simulink model "EHB_speedgoat_R2020a_V1"  (R2020a)
settings: Solver=FixedStepDiscrete  StartTime=0.0  StopTime=inf  FixedStep=0.001  RelTol=1e-3  EnableMultiTasking=on
model workspace (MAT data in the model file):
  A : Simulink.Signal (value not decoded)
  B : Simulink.Signal (value not decoded)
  C : Simulink.Signal (value not decoded)
  D : Simulink.Signal (value not decoded)
  E : Simulink.Signal (value not decoded)
  calin = [-9.96 -7.98 -5.98 -3.99 -1.994 0 1.995 3.992 5.99 7.98 9.97]
  calout = [-10 -8 -6 -4 -2 0 2 4 6 8 10]
symbols that are objects in the model workspace (value not decoded): C, D
undefined symbols (not defined in the file): Com1, none, ts_IO612
libraries: simulink x1436, xpcethercatlib x1223, yisutbxlib_utilities x256, xpcutilitieslib x156, hdlsllib x145, canmsglib x46, speedgoatlib_IO602_4 x11, speedgoatlib_IO611 x7, slrttcplib x4, CanManageLib x3, slrtlib x3, xpcseriallib x2
(part 15 of 30)

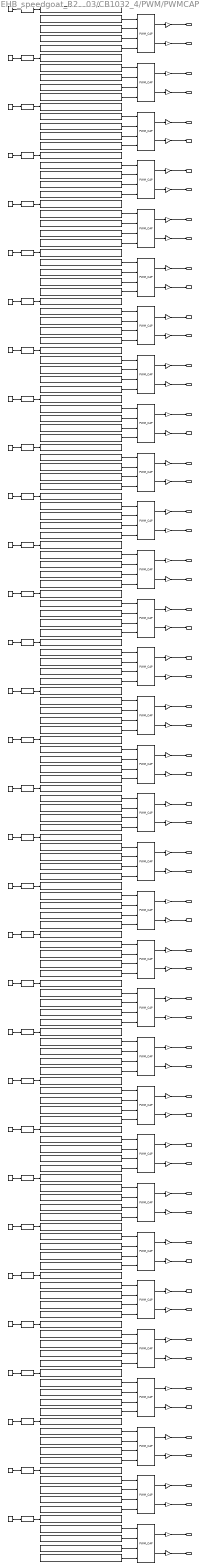
== system EHB_speedgoat_R2020a_V1/保留/TIF_03/CB1032_4/PWM/PWMCAP1 ==
  Constant CPL_CH{1..32} (32 alike) : Constant
  DTCB CPL_CH{1..32} (32 alike) : DataTypeConversion
  Gain_DC_CAP_CH{1..32} (32 alike) : Gain
  Gain_Period_CAP_CH{1..32} (32 alike) : Gain
  PDO Receive HTH_CH1 : xpcethercatlib/EtherCAT PDO Receive  Priority=2  sig_name=Box 4 (YISUWORLD_Dig).PDOGetValue process data mapping.HTH1  sig_offset=8344  sig_type=uint16  type_size=16  sig_dim=1  device_id=0  sample_time=0.001000
      settings: SourceProductBaseCode=XP
  PDO Receive HTH_CH10 : xpcethercatlib/EtherCAT PDO Receive  Priority=2  sig_name=Box 4 (YISUWORLD_Dig).PDOGetValue process data mapping.HTH10  sig_offset=8488  sig_type=uint16  type_size=16  sig_dim=1  device_id=0  sample_time=0.001000
      settings: SourceProductBaseCode=XP
  PDO Receive HTH_CH11 : xpcethercatlib/EtherCAT PDO Receive  Priority=2  sig_name=Box 4 (YISUWORLD_Dig).PDOGetValue process data mapping.HTH11  sig_offset=8504  sig_type=uint16  type_size=16  sig_dim=1  device_id=0  sample_time=0.001000
      settings: SourceProductBaseCode=XP
  PDO Receive HTH_CH12 : xpcethercatlib/EtherCAT PDO Receive  Priority=2  sig_name=Box 4 (YISUWORLD_Dig).PDOGetValue process data mapping.HTH12  sig_offset=8520  sig_type=uint16  type_size=16  sig_dim=1  device_id=0  sample_time=0.001000
      settings: SourceProductBaseCode=XP
  PDO Receive HTH_CH13 : xpcethercatlib/EtherCAT PDO Receive  Priority=2  sig_name=Box 4 (YISUWORLD_Dig).PDOGetValue process data mapping.HTH13  sig_offset=8536  sig_type=uint16  type_size=16  sig_dim=1  device_id=0  sample_time=0.001000
      settings: SourceProductBaseCode=XP
  PDO Receive HTH_CH14 : xpcethercatlib/EtherCAT PDO Receive  Priority=2  sig_name=Box 4 (YISUWORLD_Dig).PDOGetValue process data mapping.HTH14  sig_offset=8552  sig_type=uint16  type_size=16  sig_dim=1  device_id=0  sample_time=0.001000
      settings: SourceProductBaseCode=XP
  PDO Receive HTH_CH15 : xpcethercatlib/EtherCAT PDO Receive  Priority=2  sig_name=Box 4 (YISUWORLD_Dig).PDOGetValue process data mapping.HTH15  sig_offset=8568  sig_type=uint16  type_size=16  sig_dim=1  device_id=0  sample_time=0.001000
      settings: SourceProductBaseCode=XP
  PDO Receive HTH_CH16 : xpcethercatlib/EtherCAT PDO Receive  Priority=2  sig_name=Box 4 (YISUWORLD_Dig).PDOGetValue process data mapping.HTH16  sig_offset=8584  sig_type=uint16  type_size=16  sig_dim=1  device_id=0  sample_time=0.001000
      settings: SourceProductBaseCode=XP
  PDO Receive HTH_CH17 : xpcethercatlib/EtherCAT PDO Receive  Priority=2  sig_name=Box 4 (YISUWORLD_Dig).PDOGetValue process data mapping.HTH17  sig_offset=8600  sig_type=uint16  type_size=16  sig_dim=1  device_id=0  sample_time=0.001000
      settings: SourceProductBaseCode=XP
  PDO Receive HTH_CH18 : xpcethercatlib/EtherCAT PDO Receive  Priority=2  sig_name=Box 4 (YISUWORLD_Dig).PDOGetValue process data mapping.HTH18  sig_offset=8616  sig_type=uint16  type_size=16  sig_dim=1  device_id=0  sample_time=0.001000
      settings: SourceProductBaseCode=XP
  PDO Receive HTH_CH19 : xpcethercatlib/EtherCAT PDO Receive  Priority=2  sig_name=Box 4 (YISUWORLD_Dig).PDOGetValue process data mapping.HTH19  sig_offset=8632  sig_type=uint16  type_size=16  sig_dim=1  device_id=0  sample_time=0.001000
      settings: SourceProductBaseCode=XP
  PDO Receive HTH_CH2 : xpcethercatlib/EtherCAT PDO Receive  Priority=2  sig_name=Box 4 (YISUWORLD_Dig).PDOGetValue process data mapping.HTH2  sig_offset=8360  sig_type=uint16  type_size=16  sig_dim=1  device_id=0  sample_time=0.001000
      settings: SourceProductBaseCode=XP
  PDO Receive HTH_CH20 : xpcethercatlib/EtherCAT PDO Receive  Priority=2  sig_name=Box 4 (YISUWORLD_Dig).PDOGetValue process data mapping.HTH20  sig_offset=8648  sig_type=uint16  type_size=16  sig_dim=1  device_id=0  sample_time=0.001000
      settings: SourceProductBaseCode=XP
  PDO Receive HTH_CH21 : xpcethercatlib/EtherCAT PDO Receive  Priority=2  sig_name=Box 4 (YISUWORLD_Dig).PDOGetValue process data mapping.HTH21  sig_offset=8664  sig_type=uint16  type_size=16  sig_dim=1  device_id=0  sample_time=0.001000
      settings: SourceProductBaseCode=XP
  PDO Receive HTH_CH22 : xpcethercatlib/EtherCAT PDO Receive  Priority=2  sig_name=Box 4 (YISUWORLD_Dig).PDOGetValue process data mapping.HTH22  sig_offset=8680  sig_type=uint16  type_size=16  sig_dim=1  device_id=0  sample_time=0.001000
      settings: SourceProductBaseCode=XP
  PDO Receive HTH_CH23 : xpcethercatlib/EtherCAT PDO Receive  Priority=2  sig_name=Box 4 (YISUWORLD_Dig).PDOGetValue process data mapping.HTH23  sig_offset=8696  sig_type=uint16  type_size=16  sig_dim=1  device_id=0  sample_time=0.001000
      settings: SourceProductBaseCode=XP
  PDO Receive HTH_CH24 : xpcethercatlib/EtherCAT PDO Receive  Priority=2  sig_name=Box 4 (YISUWORLD_Dig).PDOGetValue process data mapping.HTH24  sig_offset=8712  sig_type=uint16  type_size=16  sig_dim=1  device_id=0  sample_time=0.001000
      settings: SourceProductBaseCode=XP
  PDO Receive HTH_CH25 : xpcethercatlib/EtherCAT PDO Receive  Priority=2  sig_name=Box 4 (YISUWORLD_Dig).PDOGetValue process data mapping.HTH25  sig_offset=8728  sig_type=uint16  type_size=16  sig_dim=1  device_id=0  sample_time=0.001000
      settings: SourceProductBaseCode=XP
  PDO Receive HTH_CH26 : xpcethercatlib/EtherCAT PDO Receive  Priority=2  sig_name=Box 4 (YISUWORLD_Dig).PDOGetValue process data mapping.HTH26  sig_offset=8744  sig_type=uint16  type_size=16  sig_dim=1  device_id=0  sample_time=0.001000
      settings: SourceProductBaseCode=XP
  PDO Receive HTH_CH27 : xpcethercatlib/EtherCAT PDO Receive  Priority=2  sig_name=Box 4 (YISUWORLD_Dig).PDOGetValue process data mapping.HTH27  sig_offset=8760  sig_type=uint16  type_size=16  sig_dim=1  device_id=0  sample_time=0.001000
      settings: SourceProductBaseCode=XP
  PDO Receive HTH_CH28 : xpcethercatlib/EtherCAT PDO Receive  Priority=2  sig_name=Box 4 (YISUWORLD_Dig).PDOGetValue process data mapping.HTH28  sig_offset=8776  sig_type=uint16  type_size=16  sig_dim=1  device_id=0  sample_time=0.001000
      settings: SourceProductBaseCode=XP
  PDO Receive HTH_CH29 : xpcethercatlib/EtherCAT PDO Receive  Priority=2  sig_name=Box 4 (YISUWORLD_Dig).PDOGetValue process data mapping.HTH29  sig_offset=8792  sig_type=uint16  type_size=16  sig_dim=1  device_id=0  sample_time=0.001000
      settings: SourceProductBaseCode=XP
  PDO Receive HTH_CH3 : xpcethercatlib/EtherCAT PDO Receive  Priority=2  sig_name=Box 4 (YISUWORLD_Dig).PDOGetValue process data mapping.HTH3  sig_offset=8376  sig_type=uint16  type_size=16  sig_dim=1  device_id=0  sample_time=0.001000
      settings: SourceProductBaseCode=XP
  PDO Receive HTH_CH30 : xpcethercatlib/EtherCAT PDO Receive  Priority=2  sig_name=Box 4 (YISUWORLD_Dig).PDOGetValue process data mapping.HTH30  sig_offset=8808  sig_type=uint16  type_size=16  sig_dim=1  device_id=0  sample_time=0.001000
      settings: SourceProductBaseCode=XP
  PDO Receive HTH_CH31 : xpcethercatlib/EtherCAT PDO Receive  Priority=2  sig_name=Box 4 (YISUWORLD_Dig).PDOGetValue process data mapping.HTH31  sig_offset=8824  sig_type=uint16  type_size=16  sig_dim=1  device_id=0  sample_time=0.001000
      settings: SourceProductBaseCode=XP
  PDO Receive HTH_CH32 : xpcethercatlib/EtherCAT PDO Receive  Priority=2  sig_name=Box 4 (YISUWORLD_Dig).PDOGetValue process data mapping.HTH32  sig_offset=8840  sig_type=uint16  type_size=16  sig_dim=1  device_id=0  sample_time=0.001000
      settings: SourceProductBaseCode=XP
  PDO Receive HTH_CH4 : xpcethercatlib/EtherCAT PDO Receive  Priority=2  sig_name=Box 4 (YISUWORLD_Dig).PDOGetValue process data mapping.HTH4  sig_offset=8392  sig_type=uint16  type_size=16  sig_dim=1  device_id=0  sample_time=0.001000
      settings: SourceProductBaseCode=XP
  PDO Receive HTH_CH5 : xpcethercatlib/EtherCAT PDO Receive  Priority=2  sig_name=Box 4 (YISUWORLD_Dig).PDOGetValue process data mapping.HTH5  sig_offset=8408  sig_type=uint16  type_size=16  sig_dim=1  device_id=0  sample_time=0.001000
      settings: SourceProductBaseCode=XP
  PDO Receive HTH_CH6 : xpcethercatlib/EtherCAT PDO Receive  Priority=2  sig_name=Box 4 (YISUWORLD_Dig).PDOGetValue process data mapping.HTH6  sig_offset=8424  sig_type=uint16  type_size=16  sig_dim=1  device_id=0  sample_time=0.001000
      settings: SourceProductBaseCode=XP
  PDO Receive HTH_CH7 : xpcethercatlib/EtherCAT PDO Receive  Priority=2  sig_name=Box 4 (YISUWORLD_Dig).PDOGetValue process data mapping.HTH7  sig_offset=8440  sig_type=uint16  type_size=16  sig_dim=1  device_id=0  sample_time=0.001000
      settings: SourceProductBaseCode=XP
  PDO Receive HTH_CH8 : xpcethercatlib/EtherCAT PDO Receive  Priority=2  sig_name=Box 4 (YISUWORLD_Dig).PDOGetValue process data mapping.HTH8  sig_offset=8456  sig_type=uint16  type_size=16  sig_dim=1  device_id=0  sample_time=0.001000
      settings: SourceProductBaseCode=XP
  PDO Receive HTH_CH9 : xpcethercatlib/EtherCAT PDO Receive  Priority=2  sig_name=Box 4 (YISUWORLD_Dig).PDOGetValue process data mapping.HTH9  sig_offset=8472  sig_type=uint16  type_size=16  sig_dim=1  device_id=0  sample_time=0.001000
      settings: SourceProductBaseCode=XP
  PDO Receive HTL_CH1 : xpcethercatlib/EtherCAT PDO Receive  Priority=2  sig_name=Box 4 (YISUWORLD_Dig).PDOGetValue process data mapping.HTL1  sig_offset=8856  sig_type=uint16  type_size=16  sig_dim=1  device_id=0  sample_time=0.001000
      settings: SourceProductBaseCode=XP
  PDO Receive HTL_CH10 : xpcethercatlib/EtherCAT PDO Receive  Priority=2  sig_name=Box 4 (YISUWORLD_Dig).PDOGetValue process data mapping.HTL10  sig_offset=9000  sig_type=uint16  type_size=16  sig_dim=1  device_id=0  sample_time=0.001000
      settings: SourceProductBaseCode=XP
  PDO Receive HTL_CH11 : xpcethercatlib/EtherCAT PDO Receive  Priority=2  sig_name=Box 4 (YISUWORLD_Dig).PDOGetValue process data mapping.HTL11  sig_offset=9016  sig_type=uint16  type_size=16  sig_dim=1  device_id=0  sample_time=0.001000
      settings: SourceProductBaseCode=XP
  PDO Receive HTL_CH12 : xpcethercatlib/EtherCAT PDO Receive  Priority=2  sig_name=Box 4 (YISUWORLD_Dig).PDOGetValue process data mapping.HTL12  sig_offset=9032  sig_type=uint16  type_size=16  sig_dim=1  device_id=0  sample_time=0.001000
      settings: SourceProductBaseCode=XP
  PDO Receive HTL_CH13 : xpcethercatlib/EtherCAT PDO Receive  Priority=2  sig_name=Box 4 (YISUWORLD_Dig).PDOGetValue process data mapping.HTL13  sig_offset=9048  sig_type=uint16  type_size=16  sig_dim=1  device_id=0  sample_time=0.001000
      settings: SourceProductBaseCode=XP
  PDO Receive HTL_CH14 : xpcethercatlib/EtherCAT PDO Receive  Priority=2  sig_name=Box 4 (YISUWORLD_Dig).PDOGetValue process data mapping.HTL14  sig_offset=9064  sig_type=uint16  type_size=16  sig_dim=1  device_id=0  sample_time=0.001000
      settings: SourceProductBaseCode=XP
  PDO Receive HTL_CH15 : xpcethercatlib/EtherCAT PDO Receive  Priority=2  sig_name=Box 4 (YISUWORLD_Dig).PDOGetValue process data mapping.HTL15  sig_offset=9080  sig_type=uint16  type_size=16  sig_dim=1  device_id=0  sample_time=0.001000
      settings: SourceProductBaseCode=XP
  PDO Receive HTL_CH16 : xpcethercatlib/EtherCAT PDO Receive  Priority=2  sig_name=Box 4 (YISUWORLD_Dig).PDOGetValue process data mapping.HTL16  sig_offset=9096  sig_type=uint16  type_size=16  sig_dim=1  device_id=0  sample_time=0.001000
      settings: SourceProductBaseCode=XP
  PDO Receive HTL_CH17 : xpcethercatlib/EtherCAT PDO Receive  Priority=2  sig_name=Box 4 (YISUWORLD_Dig).PDOGetValue process data mapping.HTL17  sig_offset=9112  sig_type=uint16  type_size=16  sig_dim=1  device_id=0  sample_time=0.001000
      settings: SourceProductBaseCode=XP
  PDO Receive HTL_CH18 : xpcethercatlib/EtherCAT PDO Receive  Priority=2  sig_name=Box 4 (YISUWORLD_Dig).PDOGetValue process data mapping.HTL18  sig_offset=9128  sig_type=uint16  type_size=16  sig_dim=1  device_id=0  sample_time=0.001000
      settings: SourceProductBaseCode=XP
  PDO Receive HTL_CH19 : xpcethercatlib/EtherCAT PDO Receive  Priority=2  sig_name=Box 4 (YISUWORLD_Dig).PDOGetValue process data mapping.HTL19  sig_offset=9144  sig_type=uint16  type_size=16  sig_dim=1  device_id=0  sample_time=0.001000
      settings: SourceProductBaseCode=XP
  PDO Receive HTL_CH2 : xpcethercatlib/EtherCAT PDO Receive  Priority=2  sig_name=Box 4 (YISUWORLD_Dig).PDOGetValue process data mapping.HTL2  sig_offset=8872  sig_type=uint16  type_size=16  sig_dim=1  device_id=0  sample_time=0.001000
      settings: SourceProductBaseCode=XP
  PDO Receive HTL_CH20 : xpcethercatlib/EtherCAT PDO Receive  Priority=2  sig_name=Box 4 (YISUWORLD_Dig).PDOGetValue process data mapping.HTL20  sig_offset=9160  sig_type=uint16  type_size=16  sig_dim=1  device_id=0  sample_time=0.001000
      settings: SourceProductBaseCode=XP
  PDO Receive HTL_CH21 : xpcethercatlib/EtherCAT PDO Receive  Priority=2  sig_name=Box 4 (YISUWORLD_Dig).PDOGetValue process data mapping.HTL21  sig_offset=9176  sig_type=uint16  type_size=16  sig_dim=1  device_id=0  sample_time=0.001000
      settings: SourceProductBaseCode=XP
  PDO Receive HTL_CH22 : xpcethercatlib/EtherCAT PDO Receive  Priority=2  sig_name=Box 4 (YISUWORLD_Dig).PDOGetValue process data mapping.HTL22  sig_offset=9192  sig_type=uint16  type_size=16  sig_dim=1  device_id=0  sample_time=0.001000
      settings: SourceProductBaseCode=XP
  PDO Receive HTL_CH23 : xpcethercatlib/EtherCAT PDO Receive  Priority=2  sig_name=Box 4 (YISUWORLD_Dig).PDOGetValue process data mapping.HTL23  sig_offset=9208  sig_type=uint16  type_size=16  sig_dim=1  device_id=0  sample_time=0.001000
      settings: SourceProductBaseCode=XP
  PDO Receive HTL_CH24 : xpcethercatlib/EtherCAT PDO Receive  Priority=2  sig_name=Box 4 (YISUWORLD_Dig).PDOGetValue process data mapping.HTL24  sig_offset=9224  sig_type=uint16  type_size=16  sig_dim=1  device_id=0  sample_time=0.001000
      settings: SourceProductBaseCode=XP
  PDO Receive HTL_CH25 : xpcethercatlib/EtherCAT PDO Receive  Priority=2  sig_name=Box 4 (YISUWORLD_Dig).PDOGetValue process data mapping.HTL25  sig_offset=9240  sig_type=uint16  type_size=16  sig_dim=1  device_id=0  sample_time=0.001000
      settings: SourceProductBaseCode=XP
  PDO Receive HTL_CH26 : xpcethercatlib/EtherCAT PDO Receive  Priority=2  sig_name=Box 4 (YISUWORLD_Dig).PDOGetValue process data mapping.HTL26  sig_offset=9256  sig_type=uint16  type_size=16  sig_dim=1  device_id=0  sample_time=0.001000
      settings: SourceProductBaseCode=XP
  PDO Receive HTL_CH27 : xpcethercatlib/EtherCAT PDO Receive  Priority=2  sig_name=Box 4 (YISUWORLD_Dig).PDOGetValue process data mapping.HTL27  sig_offset=9272  sig_type=uint16  type_size=16  sig_dim=1  device_id=0  sample_time=0.001000
      settings: SourceProductBaseCode=XP
  PDO Receive HTL_CH28 : xpcethercatlib/EtherCAT PDO Receive  Priority=2  sig_name=Box 4 (YISUWORLD_Dig).PDOGetValue process data mapping.HTL28  sig_offset=9288  sig_type=uint16  type_size=16  sig_dim=1  device_id=0  sample_time=0.001000
      settings: SourceProductBaseCode=XP
  PDO Receive HTL_CH29 : xpcethercatlib/EtherCAT PDO Receive  Priority=2  sig_name=Box 4 (YISUWORLD_Dig).PDOGetValue process data mapping.HTL29  sig_offset=9304  sig_type=uint16  type_size=16  sig_dim=1  device_id=0  sample_time=0.001000
      settings: SourceProductBaseCode=XP
  PDO Receive HTL_CH3 : xpcethercatlib/EtherCAT PDO Receive  Priority=2  sig_name=Box 4 (YISUWORLD_Dig).PDOGetValue process data mapping.HTL3  sig_offset=8888  sig_type=uint16  type_size=16  sig_dim=1  device_id=0  sample_time=0.001000
      settings: SourceProductBaseCode=XP
  PDO Receive HTL_CH30 : xpcethercatlib/EtherCAT PDO Receive  Priority=2  sig_name=Box 4 (YISUWORLD_Dig).PDOGetValue process data mapping.HTL30  sig_offset=9320  sig_type=uint16  type_size=16  sig_dim=1  device_id=0  sample_time=0.001000
      settings: SourceProductBaseCode=XP
  PDO Receive HTL_CH31 : xpcethercatlib/EtherCAT PDO Receive  Priority=2  sig_name=Box 4 (YISUWORLD_Dig).PDOGetValue process data mapping.HTL31  sig_offset=9336  sig_type=uint16  type_size=16  sig_dim=1  device_id=0  sample_time=0.001000
      settings: SourceProductBaseCode=XP
  PDO Receive HTL_CH32 : xpcethercatlib/EtherCAT PDO Receive  Priority=2  sig_name=Box 4 (YISUWORLD_Dig).PDOGetValue process data mapping.HTL32  sig_offset=9352  sig_type=uint16  type_size=16  sig_dim=1  device_id=0  sample_time=0.001000
      settings: SourceProductBaseCode=XP
  PDO Receive HTL_CH4 : xpcethercatlib/EtherCAT PDO Receive  Priority=2  sig_name=Box 4 (YISUWORLD_Dig).PDOGetValue process data mapping.HTL4  sig_offset=8904  sig_type=uint16  type_size=16  sig_dim=1  device_id=0  sample_time=0.001000
      settings: SourceProductBaseCode=XP
  PDO Receive HTL_CH5 : xpcethercatlib/EtherCAT PDO Receive  Priority=2  sig_name=Box 4 (YISUWORLD_Dig).PDOGetValue process data mapping.HTL5  sig_offset=8920  sig_type=uint16  type_size=16  sig_dim=1  device_id=0  sample_time=0.001000
      settings: SourceProductBaseCode=XP
  PDO Receive HTL_CH6 : xpcethercatlib/EtherCAT PDO Receive  Priority=2  sig_name=Box 4 (YISUWORLD_Dig).PDOGetValue process data mapping.HTL6  sig_offset=8936  sig_type=uint16  type_size=16  sig_dim=1  device_id=0  sample_time=0.001000
      settings: SourceProductBaseCode=XP
  PDO Receive HTL_CH7 : xpcethercatlib/EtherCAT PDO Receive  Priority=2  sig_name=Box 4 (YISUWORLD_Dig).PDOGetValue process data mapping.HTL7  sig_offset=8952  sig_type=uint16  type_size=16  sig_dim=1  device_id=0  sample_time=0.001000
      settings: SourceProductBaseCode=XP
  PDO Receive HTL_CH8 : xpcethercatlib/EtherCAT PDO Receive  Priority=2  sig_name=Box 4 (YISUWORLD_Dig).PDOGetValue process data mapping.HTL8  sig_offset=8968  sig_type=uint16  type_size=16  sig_dim=1  device_id=0  sample_time=0.001000
      settings: SourceProductBaseCode=XP
  PDO Receive HTL_CH9 : xpcethercatlib/EtherCAT PDO Receive  Priority=2  sig_name=Box 4 (YISUWORLD_Dig).PDOGetValue process data mapping.HTL9  sig_offset=8984  sig_type=uint16  type_size=16  sig_dim=1  device_id=0  sample_time=0.001000
      settings: SourceProductBaseCode=XP
  PDO Receive PH_CH1 : xpcethercatlib/EtherCAT PDO Receive  Priority=2  sig_name=Box 4 (YISUWORLD_Dig).PDOGetValue process data mapping.PH1  sig_offset=9368  sig_type=uint16  type_size=16  sig_dim=1  device_id=0  sample_time=0.001000
      settings: SourceProductBaseCode=XP
  PDO Receive PH_CH10 : xpcethercatlib/EtherCAT PDO Receive  Priority=2  sig_name=Box 4 (YISUWORLD_Dig).PDOGetValue process data mapping.PH10  sig_offset=9512  sig_type=uint16  type_size=16  sig_dim=1  device_id=0  sample_time=0.001000
      settings: SourceProductBaseCode=XP
  PDO Receive PH_CH11 : xpcethercatlib/EtherCAT PDO Receive  Priority=2  sig_name=Box 4 (YISUWORLD_Dig).PDOGetValue process data mapping.PH11  sig_offset=9528  sig_type=uint16  type_size=16  sig_dim=1  device_id=0  sample_time=0.001000
      settings: SourceProductBaseCode=XP
  PDO Receive PH_CH12 : xpcethercatlib/EtherCAT PDO Receive  Priority=2  sig_name=Box 4 (YISUWORLD_Dig).PDOGetValue process data mapping.PH12  sig_offset=9544  sig_type=uint16  type_size=16  sig_dim=1  device_id=0  sample_time=0.001000
      settings: SourceProductBaseCode=XP
  PDO Receive PH_CH13 : xpcethercatlib/EtherCAT PDO Receive  Priority=2  sig_name=Box 4 (YISUWORLD_Dig).PDOGetValue process data mapping.PH13  sig_offset=9560  sig_type=uint16  type_size=16  sig_dim=1  device_id=0  sample_time=0.001000
      settings: SourceProductBaseCode=XP
  PDO Receive PH_CH14 : xpcethercatlib/EtherCAT PDO Receive  Priority=2  sig_name=Box 4 (YISUWORLD_Dig).PDOGetValue process data mapping.PH14  sig_offset=9576  sig_type=uint16  type_size=16  sig_dim=1  device_id=0  sample_time=0.001000
      settings: SourceProductBaseCode=XP
  PDO Receive PH_CH15 : xpcethercatlib/EtherCAT PDO Receive  Priority=2  sig_name=Box 4 (YISUWORLD_Dig).PDOGetValue process data mapping.PH15  sig_offset=9592  sig_type=uint16  type_size=16  sig_dim=1  device_id=0  sample_time=0.001000
      settings: SourceProductBaseCode=XP
  PDO Receive PH_CH16 : xpcethercatlib/EtherCAT PDO Receive  Priority=2  sig_name=Box 4 (YISUWORLD_Dig).PDOGetValue process data mapping.PH16  sig_offset=9608  sig_type=uint16  type_size=16  sig_dim=1  device_id=0  sample_time=0.001000
      settings: SourceProductBaseCode=XP
  PDO Receive PH_CH17 : xpcethercatlib/EtherCAT PDO Receive  Priority=2  sig_name=Box 4 (YISUWORLD_Dig).PDOGetValue process data mapping.PH17  sig_offset=9624  sig_type=uint16  type_size=16  sig_dim=1  device_id=0  sample_time=0.001000
      settings: SourceProductBaseCode=XP
  PDO Receive PH_CH18 : xpcethercatlib/EtherCAT PDO Receive  Priority=2  sig_name=Box 4 (YISUWORLD_Dig).PDOGetValue process data mapping.PH18  sig_offset=9640  sig_type=uint16  type_size=16  sig_dim=1  device_id=0  sample_time=0.001000
      settings: SourceProductBaseCode=XP
  PDO Receive PH_CH19 : xpcethercatlib/EtherCAT PDO Receive  Priority=2  sig_name=Box 4 (YISUWORLD_Dig).PDOGetValue process data mapping.PH19  sig_offset=9656  sig_type=uint16  type_size=16  sig_dim=1  device_id=0  sample_time=0.001000
      settings: SourceProductBaseCode=XP
  PDO Receive PH_CH2 : xpcethercatlib/EtherCAT PDO Receive  Priority=2  sig_name=Box 4 (YISUWORLD_Dig).PDOGetValue process data mapping.PH2  sig_offset=9384  sig_type=uint16  type_size=16  sig_dim=1  device_id=0  sample_time=0.001000
      settings: SourceProductBaseCode=XP
  PDO Receive PH_CH20 : xpcethercatlib/EtherCAT PDO Receive  Priority=2  sig_name=Box 4 (YISUWORLD_Dig).PDOGetValue process data mapping.PH20  sig_offset=9672  sig_type=uint16  type_size=16  sig_dim=1  device_id=0  sample_time=0.001000
      settings: SourceProductBaseCode=XP
  PDO Receive PH_CH21 : xpcethercatlib/EtherCAT PDO Receive  Priority=2  sig_name=Box 4 (YISUWORLD_Dig).PDOGetValue process data mapping.PH21  sig_offset=9688  sig_type=uint16  type_size=16  sig_dim=1  device_id=0  sample_time=0.001000
      settings: SourceProductBaseCode=XP
  PDO Receive PH_CH22 : xpcethercatlib/EtherCAT PDO Receive  Priority=2  sig_name=Box 4 (YISUWORLD_Dig).PDOGetValue process data mapping.PH22  sig_offset=9704  sig_type=uint16  type_size=16  sig_dim=1  device_id=0  sample_time=0.001000
      settings: SourceProductBaseCode=XP
  PDO Receive PH_CH23 : xpcethercatlib/EtherCAT PDO Receive  Priority=2  sig_name=Box 4 (YISUWORLD_Dig).PDOGetValue process data mapping.PH23  sig_offset=9720  sig_type=uint16  type_size=16  sig_dim=1  device_id=0  sample_time=0.001000
      settings: SourceProductBaseCode=XP
  PDO Receive PH_CH24 : xpcethercatlib/EtherCAT PDO Receive  Priority=2  sig_name=Box 4 (YISUWORLD_Dig).PDOGetValue process data mapping.PH24  sig_offset=9736  sig_type=uint16  type_size=16  sig_dim=1  device_id=0  sample_time=0.001000
      settings: SourceProductBaseCode=XP
  PDO Receive PH_CH25 : xpcethercatlib/EtherCAT PDO Receive  Priority=2  sig_name=Box 4 (YISUWORLD_Dig).PDOGetValue process data mapping.PH25  sig_offset=9752  sig_type=uint16  type_size=16  sig_dim=1  device_id=0  sample_time=0.001000
      settings: SourceProductBaseCode=XP
  PDO Receive PH_CH26 : xpcethercatlib/EtherCAT PDO Receive  Priority=2  sig_name=Box 4 (YISUWORLD_Dig).PDOGetValue process data mapping.PH26  sig_offset=9768  sig_type=uint16  type_size=16  sig_dim=1  device_id=0  sample_time=0.001000
      settings: SourceProductBaseCode=XP
  PDO Receive PH_CH27 : xpcethercatlib/EtherCAT PDO Receive  Priority=2  sig_name=Box 4 (YISUWORLD_Dig).PDOGetValue process data mapping.PH27  sig_offset=9784  sig_type=uint16  type_size=16  sig_dim=1  device_id=0  sample_time=0.001000
      settings: SourceProductBaseCode=XP
  PDO Receive PH_CH28 : xpcethercatlib/EtherCAT PDO Receive  Priority=2  sig_name=Box 4 (YISUWORLD_Dig).PDOGetValue process data mapping.PH28  sig_offset=9800  sig_type=uint16  type_size=16  sig_dim=1  device_id=0  sample_time=0.001000
      settings: SourceProductBaseCode=XP
  PDO Receive PH_CH29 : xpcethercatlib/EtherCAT PDO Receive  Priority=2  sig_name=Box 4 (YISUWORLD_Dig).PDOGetValue process data mapping.PH29  sig_offset=9816  sig_type=uint16  type_size=16  sig_dim=1  device_id=0  sample_time=0.001000
      settings: SourceProductBaseCode=XP
  PDO Receive PH_CH3 : xpcethercatlib/EtherCAT PDO Receive  Priority=2  sig_name=Box 4 (YISUWORLD_Dig).PDOGetValue process data mapping.PH3  sig_offset=9400  sig_type=uint16  type_size=16  sig_dim=1  device_id=0  sample_time=0.001000
      settings: SourceProductBaseCode=XP
  PDO Receive PH_CH30 : xpcethercatlib/EtherCAT PDO Receive  Priority=2  sig_name=Box 4 (YISUWORLD_Dig).PDOGetValue process data mapping.PH30  sig_offset=9832  sig_type=uint16  type_size=16  sig_dim=1  device_id=0  sample_time=0.001000
      settings: SourceProductBaseCode=XP
  PDO Receive PH_CH31 : xpcethercatlib/EtherCAT PDO Receive  Priority=2  sig_name=Box 4 (YISUWORLD_Dig).PDOGetValue process data mapping.PH31  sig_offset=9848  sig_type=uint16  type_size=16  sig_dim=1  device_id=0  sample_time=0.001000
      settings: SourceProductBaseCode=XP
  PDO Receive PH_CH32 : xpcethercatlib/EtherCAT PDO Receive  Priority=2  sig_name=Box 4 (YISUWORLD_Dig).PDOGetValue process data mapping.PH32  sig_offset=9864  sig_type=uint16  type_size=16  sig_dim=1  device_id=0  sample_time=0.001000
      settings: SourceProductBaseCode=XP
  PDO Receive PH_CH4 : xpcethercatlib/EtherCAT PDO Receive  Priority=2  sig_name=Box 4 (YISUWORLD_Dig).PDOGetValue process data mapping.PH4  sig_offset=9416  sig_type=uint16  type_size=16  sig_dim=1  device_id=0  sample_time=0.001000
      settings: SourceProductBaseCode=XP
  PDO Receive PH_CH5 : xpcethercatlib/EtherCAT PDO Receive  Priority=2  sig_name=Box 4 (YISUWORLD_Dig).PDOGetValue process data mapping.PH5  sig_offset=9432  sig_type=uint16  type_size=16  sig_dim=1  device_id=0  sample_time=0.001000
      settings: SourceProductBaseCode=XP
  PDO Receive PH_CH6 : xpcethercatlib/EtherCAT PDO Receive  Priority=2  sig_name=Box 4 (YISUWORLD_Dig).PDOGetValue process data mapping.PH6  sig_offset=9448  sig_type=uint16  type_size=16  sig_dim=1  device_id=0  sample_time=0.001000
      settings: SourceProductBaseCode=XP
  PDO Receive PH_CH7 : xpcethercatlib/EtherCAT PDO Receive  Priority=2  sig_name=Box 4 (YISUWORLD_Dig).PDOGetValue process data mapping.PH7  sig_offset=9464  sig_type=uint16  type_size=16  sig_dim=1  device_id=0  sample_time=0.001000
      settings: SourceProductBaseCode=XP
  PDO Receive PH_CH8 : xpcethercatlib/EtherCAT PDO Receive  Priority=2  sig_name=Box 4 (YISUWORLD_Dig).PDOGetValue process data mapping.PH8  sig_offset=9480  sig_type=uint16  type_size=16  sig_dim=1  device_id=0  sample_time=0.001000
      settings: SourceProductBaseCode=XP
  PDO Receive PH_CH9 : xpcethercatlib/EtherCAT PDO Receive  Priority=2  sig_name=Box 4 (YISUWORLD_Dig).PDOGetValue process data mapping.PH9  sig_offset=9496  sig_type=uint16  type_size=16  sig_dim=1  device_id=0  sample_time=0.001000
      settings: SourceProductBaseCode=XP
  PDO Receive PL_CH1 : xpcethercatlib/EtherCAT PDO Receive  Priority=2  sig_name=Box 4 (YISUWORLD_Dig).PDOGetValue process data mapping.PL1  sig_offset=9880  sig_type=uint16  type_size=16  sig_dim=1  device_id=0  sample_time=0.001000
      settings: SourceProductBaseCode=XP
  PDO Receive PL_CH10 : xpcethercatlib/EtherCAT PDO Receive  Priority=2  sig_name=Box 4 (YISUWORLD_Dig).PDOGetValue process data mapping.PL10  sig_offset=10024  sig_type=uint16  type_size=16  sig_dim=1  device_id=0  sample_time=0.001000
      settings: SourceProductBaseCode=XP
  PDO Receive PL_CH11 : xpcethercatlib/EtherCAT PDO Receive  Priority=2  sig_name=Box 4 (YISUWORLD_Dig).PDOGetValue process data mapping.PL11  sig_offset=10040  sig_type=uint16  type_size=16  sig_dim=1  device_id=0  sample_time=0.001000
      settings: SourceProductBaseCode=XP
  PDO Receive PL_CH12 : xpcethercatlib/EtherCAT PDO Receive  Priority=2  sig_name=Box 4 (YISUWORLD_Dig).PDOGetValue process data mapping.PL12  sig_offset=10056  sig_type=uint16  type_size=16  sig_dim=1  device_id=0  sample_time=0.001000
      settings: SourceProductBaseCode=XP
  PDO Receive PL_CH13 : xpcethercatlib/EtherCAT PDO Receive  Priority=2  sig_name=Box 4 (YISUWORLD_Dig).PDOGetValue process data mapping.PL13  sig_offset=10072  sig_type=uint16  type_size=16  sig_dim=1  device_id=0  sample_time=0.001000
      settings: SourceProductBaseCode=XP
  PDO Receive PL_CH14 : xpcethercatlib/EtherCAT PDO Receive  Priority=2  sig_name=Box 4 (YISUWORLD_Dig).PDOGetValue process data mapping.PL14  sig_offset=10088  sig_type=uint16  type_size=16  sig_dim=1  device_id=0  sample_time=0.001000
      settings: SourceProductBaseCode=XP
  PDO Receive PL_CH15 : xpcethercatlib/EtherCAT PDO Receive  Priority=2  sig_name=Box 4 (YISUWORLD_Dig).PDOGetValue process data mapping.PL15  sig_offset=10104  sig_type=uint16  type_size=16  sig_dim=1  device_id=0  sample_time=0.001000
      settings: SourceProductBaseCode=XP
  PDO Receive PL_CH16 : xpcethercatlib/EtherCAT PDO Receive  Priority=2  sig_name=Box 4 (YISUWORLD_Dig).PDOGetValue process data mapping.PL16  sig_offset=10120  sig_type=uint16  type_size=16  sig_dim=1  device_id=0  sample_time=0.001000
      settings: SourceProductBaseCode=XP
  PDO Receive PL_CH17 : xpcethercatlib/EtherCAT PDO Receive  Priority=2  sig_name=Box 4 (YISUWORLD_Dig).PDOGetValue process data mapping.PL17  sig_offset=10136  sig_type=uint16  type_size=16  sig_dim=1  device_id=0  sample_time=0.001000
      settings: SourceProductBaseCode=XP
  PDO Receive PL_CH18 : xpcethercatlib/EtherCAT PDO Receive  Priority=2  sig_name=Box 4 (YISUWORLD_Dig).PDOGetValue process data mapping.PL18  sig_offset=10152  sig_type=uint16  type_size=16  sig_dim=1  device_id=0  sample_time=0.001000
      settings: SourceProductBaseCode=XP
  PDO Receive PL_CH19 : xpcethercatlib/EtherCAT PDO Receive  Priority=2  sig_name=Box 4 (YISUWORLD_Dig).PDOGetValue process data mapping.PL19  sig_offset=10168  sig_type=uint16  type_size=16  sig_dim=1  device_id=0  sample_time=0.001000
      settings: SourceProductBaseCode=XP
  PDO Receive PL_CH2 : xpcethercatlib/EtherCAT PDO Receive  Priority=2  sig_name=Box 4 (YISUWORLD_Dig).PDOGetValue process data mapping.PL2  sig_offset=9896  sig_type=uint16  type_size=16  sig_dim=1  device_id=0  sample_time=0.001000
      settings: SourceProductBaseCode=XP
  PDO Receive PL_CH20 : xpcethercatlib/EtherCAT PDO Receive  Priority=2  sig_name=Box 4 (YISUWORLD_Dig).PDOGetValue process data mapping.PL20  sig_offset=10184  sig_type=uint16  type_size=16  sig_dim=1  device_id=0  sample_time=0.001000
      settings: SourceProductBaseCode=XP
  PDO Receive PL_CH21 : xpcethercatlib/EtherCAT PDO Receive  Priority=2  sig_name=Box 4 (YISUWORLD_Dig).PDOGetValue process data mapping.PL21  sig_offset=10200  sig_type=uint16  type_size=16  sig_dim=1  device_id=0  sample_time=0.001000
      settings: SourceProductBaseCode=XP
  PDO Receive PL_CH22 : xpcethercatlib/EtherCAT PDO Receive  Priority=2  sig_name=Box 4 (YISUWORLD_Dig).PDOGetValue process data mapping.PL22  sig_offset=10216  sig_type=uint16  type_size=16  sig_dim=1  device_id=0  sample_time=0.001000
      settings: SourceProductBaseCode=XP
  PDO Receive PL_CH23 : xpcethercatlib/EtherCAT PDO Receive  Priority=2  sig_name=Box 4 (YISUWORLD_Dig).PDOGetValue process data mapping.PL23  sig_offset=10232  sig_type=uint16  type_size=16  sig_dim=1  device_id=0  sample_time=0.001000
      settings: SourceProductBaseCode=XP
  PDO Receive PL_CH24 : xpcethercatlib/EtherCAT PDO Receive  Priority=2  sig_name=Box 4 (YISUWORLD_Dig).PDOGetValue process data mapping.PL24  sig_offset=10248  sig_type=uint16  type_size=16  sig_dim=1  device_id=0  sample_time=0.001000
      settings: SourceProductBaseCode=XP
  PDO Receive PL_CH25 : xpcethercatlib/EtherCAT PDO Receive  Priority=2  sig_name=Box 4 (YISUWORLD_Dig).PDOGetValue process data mapping.PL25  sig_offset=10264  sig_type=uint16  type_size=16  sig_dim=1  device_id=0  sample_time=0.001000
      settings: SourceProductBaseCode=XP
  PDO Receive PL_CH26 : xpcethercatlib/EtherCAT PDO Receive  Priority=2  sig_name=Box 4 (YISUWORLD_Dig).PDOGetValue process data mapping.PL26  sig_offset=10280  sig_type=uint16  type_size=16  sig_dim=1  device_id=0  sample_time=0.001000
      settings: SourceProductBaseCode=XP
  PDO Receive PL_CH27 : xpcethercatlib/EtherCAT PDO Receive  Priority=2  sig_name=Box 4 (YISUWORLD_Dig).PDOGetValue process data mapping.PL27  sig_offset=10296  sig_type=uint16  type_size=16  sig_dim=1  device_id=0  sample_time=0.001000
      settings: SourceProductBaseCode=XP
  PDO Receive PL_CH28 : xpcethercatlib/EtherCAT PDO Receive  Priority=2  sig_name=Box 4 (YISUWORLD_Dig).PDOGetValue process data mapping.PL28  sig_offset=10312  sig_type=uint16  type_size=16  sig_dim=1  device_id=0  sample_time=0.001000
      settings: SourceProductBaseCode=XP
  PDO Receive PL_CH29 : xpcethercatlib/EtherCAT PDO Receive  Priority=2  sig_name=Box 4 (YISUWORLD_Dig).PDOGetValue process data mapping.PL29  sig_offset=10328  sig_type=uint16  type_size=16  sig_dim=1  device_id=0  sample_time=0.001000
      settings: SourceProductBaseCode=XP
  PDO Receive PL_CH3 : xpcethercatlib/EtherCAT PDO Receive  Priority=2  sig_name=Box 4 (YISUWORLD_Dig).PDOGetValue process data mapping.PL3  sig_offset=9912  sig_type=uint16  type_size=16  sig_dim=1  device_id=0  sample_time=0.001000
      settings: SourceProductBaseCode=XP
  PDO Receive PL_CH30 : xpcethercatlib/EtherCAT PDO Receive  Priority=2  sig_name=Box 4 (YISUWORLD_Dig).PDOGetValue process data mapping.PL30  sig_offset=10344  sig_type=uint16  type_size=16  sig_dim=1  device_id=0  sample_time=0.001000
      settings: SourceProductBaseCode=XP
  PDO Receive PL_CH31 : xpcethercatlib/EtherCAT PDO Receive  Priority=2  sig_name=Box 4 (YISUWORLD_Dig).PDOGetValue process data mapping.PL31  sig_offset=10360  sig_type=uint16  type_size=16  sig_dim=1  device_id=0  sample_time=0.001000
      settings: SourceProductBaseCode=XP
  PDO Receive PL_CH32 : xpcethercatlib/EtherCAT PDO Receive  Priority=2  sig_name=Box 4 (YISUWORLD_Dig).PDOGetValue process data mapping.PL32  sig_offset=10376  sig_type=uint16  type_size=16  sig_dim=1  device_id=0  sample_time=0.001000
      settings: SourceProductBaseCode=XP
  PDO Receive PL_CH4 : xpcethercatlib/EtherCAT PDO Receive  Priority=2  sig_name=Box 4 (YISUWORLD_Dig).PDOGetValue process data mapping.PL4  sig_offset=9928  sig_type=uint16  type_size=16  sig_dim=1  device_id=0  sample_time=0.001000
      settings: SourceProductBaseCode=XP
  PDO Receive PL_CH5 : xpcethercatlib/EtherCAT PDO Receive  Priority=2  sig_name=Box 4 (YISUWORLD_Dig).PDOGetValue process data mapping.PL5  sig_offset=9944  sig_type=uint16  type_size=16  sig_dim=1  device_id=0  sample_time=0.001000
      settings: SourceProductBaseCode=XP
  PDO Receive PL_CH6 : xpcethercatlib/EtherCAT PDO Receive  Priority=2  sig_name=Box 4 (YISUWORLD_Dig).PDOGetValue process data mapping.PL6  sig_offset=9960  sig_type=uint16  type_size=16  sig_dim=1  device_id=0  sample_time=0.001000
      settings: SourceProductBaseCode=XP
  PDO Receive PL_CH7 : xpcethercatlib/EtherCAT PDO Receive  Priority=2  sig_name=Box 4 (YISUWORLD_Dig).PDOGetValue process data mapping.PL7  sig_offset=9976  sig_type=uint16  type_size=16  sig_dim=1  device_id=0  sample_time=0.001000
      settings: SourceProductBaseCode=XP
  PDO Receive PL_CH8 : xpcethercatlib/EtherCAT PDO Receive  Priority=2  sig_name=Box 4 (YISUWORLD_Dig).PDOGetValue process data mapping.PL8  sig_offset=9992  sig_type=uint16  type_size=16  sig_dim=1  device_id=0  sample_time=0.001000
      settings: SourceProductBaseCode=XP
  PDO Receive PL_CH9 : xpcethercatlib/EtherCAT PDO Receive  Priority=2  sig_name=Box 4 (YISUWORLD_Dig).PDOGetValue process data mapping.PL9  sig_offset=10008  sig_type=uint16  type_size=16  sig_dim=1  device_id=0  sample_time=0.001000
      settings: SourceProductBaseCode=XP
  PDO Transmit CPL_CH1 : xpcethercatlib/EtherCAT PDO Transmit   Priority=3  sig_name=Box 4 (YISUWORLD_Dig).PDOSet1 process data mapping.CPL1  sig_offset=10296  sig_type=uint16  type_size=16  sig_dim=1  device_id=0  sample_time=0.001000
      settings: SourceProductBaseCode=XP
  PDO Transmit CPL_CH10 : xpcethercatlib/EtherCAT PDO Transmit   Priority=3  sig_name=Box 4 (YISUWORLD_Dig).PDOSet1 process data mapping.CPL10  sig_offset=10440  sig_type=uint16  type_size=16  sig_dim=1  device_id=0  sample_time=0.001000
      settings: SourceProductBaseCode=XP
  PDO Transmit CPL_CH11 : xpcethercatlib/EtherCAT PDO Transmit   Priority=3  sig_name=Box 4 (YISUWORLD_Dig).PDOSet1 process data mapping.CPL11  sig_offset=10456  sig_type=uint16  type_size=16  sig_dim=1  device_id=0  sample_time=0.001000
      settings: SourceProductBaseCode=XP
  PDO Transmit CPL_CH12 : xpcethercatlib/EtherCAT PDO Transmit   Priority=3  sig_name=Box 4 (YISUWORLD_Dig).PDOSet1 process data mapping.CPL12  sig_offset=10472  sig_type=uint16  type_size=16  sig_dim=1  device_id=0  sample_time=0.001000
      settings: SourceProductBaseCode=XP
  PDO Transmit CPL_CH13 : xpcethercatlib/EtherCAT PDO Transmit   Priority=3  sig_name=Box 4 (YISUWORLD_Dig).PDOSet1 process data mapping.CPL13  sig_offset=10488  sig_type=uint16  type_size=16  sig_dim=1  device_id=0  sample_time=0.001000
      settings: SourceProductBaseCode=XP
  PDO Transmit CPL_CH14 : xpcethercatlib/EtherCAT PDO Transmit   Priority=3  sig_name=Box 4 (YISUWORLD_Dig).PDOSet1 process data mapping.CPL14  sig_offset=10504  sig_type=uint16  type_size=16  sig_dim=1  device_id=0  sample_time=0.001000
      settings: SourceProductBaseCode=XP
  PDO Transmit CPL_CH15 : xpcethercatlib/EtherCAT PDO Transmit   Priority=3  sig_name=Box 4 (YISUWORLD_Dig).PDOSet1 process data mapping.CPL15  sig_offset=10520  sig_type=uint16  type_size=16  sig_dim=1  device_id=0  sample_time=0.001000
      settings: SourceProductBaseCode=XP
  PDO Transmit CPL_CH16 : xpcethercatlib/EtherCAT PDO Transmit   Priority=3  sig_name=Box 4 (YISUWORLD_Dig).PDOSet1 process data mapping.CPL16  sig_offset=10536  sig_type=uint16  type_size=16  sig_dim=1  device_id=0  sample_time=0.001000
      settings: SourceProductBaseCode=XP
  PDO Transmit CPL_CH17 : xpcethercatlib/EtherCAT PDO Transmit   Priority=3  sig_name=Box 4 (YISUWORLD_Dig).PDOSet1 process data mapping.CPL17  sig_offset=10552  sig_type=uint16  type_size=16  sig_dim=1  device_id=0  sample_time=0.001000
      settings: SourceProductBaseCode=XP
  PDO Transmit CPL_CH18 : xpcethercatlib/EtherCAT PDO Transmit   Priority=3  sig_name=Box 4 (YISUWORLD_Dig).PDOSet1 process data mapping.CPL18  sig_offset=10568  sig_type=uint16  type_size=16  sig_dim=1  device_id=0  sample_time=0.001000
      settings: SourceProductBaseCode=XP
  PDO Transmit CPL_CH19 : xpcethercatlib/EtherCAT PDO Transmit   Priority=3  sig_name=Box 4 (YISUWORLD_Dig).PDOSet1 process data mapping.CPL19  sig_offset=10584  sig_type=uint16  type_size=16  sig_dim=1  device_id=0  sample_time=0.001000
      settings: SourceProductBaseCode=XP
  PDO Transmit CPL_CH2 : xpcethercatlib/EtherCAT PDO Transmit   Priority=3  sig_name=Box 4 (YISUWORLD_Dig).PDOSet1 process data mapping.CPL2  sig_offset=10312  sig_type=uint16  type_size=16  sig_dim=1  device_id=0  sample_time=0.001000
      settings: SourceProductBaseCode=XP
  PDO Transmit CPL_CH20 : xpcethercatlib/EtherCAT PDO Transmit   Priority=3  sig_name=Box 4 (YISUWORLD_Dig).PDOSet1 process data mapping.CPL20  sig_offset=10600  sig_type=uint16  type_size=16  sig_dim=1  device_id=0  sample_time=0.001000
      settings: SourceProductBaseCode=XP
  PDO Transmit CPL_CH21 : xpcethercatlib/EtherCAT PDO Transmit   Priority=3  sig_name=Box 4 (YISUWORLD_Dig).PDOSet1 process data mapping.CPL21  sig_offset=10616  sig_type=uint16  type_size=16  sig_dim=1  device_id=0  sample_time=0.001000
      settings: SourceProductBaseCode=XP
  PDO Transmit CPL_CH22 : xpcethercatlib/EtherCAT PDO Transmit   Priority=3  sig_name=Box 4 (YISUWORLD_Dig).PDOSet1 process data mapping.CPL22  sig_offset=10632  sig_type=uint16  type_size=16  sig_dim=1  device_id=0  sample_time=0.001000
      settings: SourceProductBaseCode=XP
  PDO Transmit CPL_CH23 : xpcethercatlib/EtherCAT PDO Transmit   Priority=3  sig_name=Box 4 (YISUWORLD_Dig).PDOSet1 process data mapping.CPL23  sig_offset=10648  sig_type=uint16  type_size=16  sig_dim=1  device_id=0  sample_time=0.001000
      settings: SourceProductBaseCode=XP
  PDO Transmit CPL_CH24 : xpcethercatlib/EtherCAT PDO Transmit   Priority=3  sig_name=Box 4 (YISUWORLD_Dig).PDOSet1 process data mapping.CPL24  sig_offset=10664  sig_type=uint16  type_size=16  sig_dim=1  device_id=0  sample_time=0.001000
      settings: SourceProductBaseCode=XP
  PDO Transmit CPL_CH25 : xpcethercatlib/EtherCAT PDO Transmit   Priority=3  sig_name=Box 4 (YISUWORLD_Dig).PDOSet1 process data mapping.CPL25  sig_offset=10680  sig_type=uint16  type_size=16  sig_dim=1  device_id=0  sample_time=0.001000
      settings: SourceProductBaseCode=XP
  PDO Transmit CPL_CH26 : xpcethercatlib/EtherCAT PDO Transmit   Priority=3  sig_name=Box 4 (YISUWORLD_Dig).PDOSet1 process data mapping.CPL26  sig_offset=10696  sig_type=uint16  type_size=16  sig_dim=1  device_id=0  sample_time=0.001000
      settings: SourceProductBaseCode=XP
  PDO Transmit CPL_CH27 : xpcethercatlib/EtherCAT PDO Transmit   Priority=3  sig_name=Box 4 (YISUWORLD_Dig).PDOSet1 process data mapping.CPL27  sig_offset=10712  sig_type=uint16  type_size=16  sig_dim=1  device_id=0  sample_time=0.001000
      settings: SourceProductBaseCode=XP
  PDO Transmit CPL_CH28 : xpcethercatlib/EtherCAT PDO Transmit   Priority=3  sig_name=Box 4 (YISUWORLD_Dig).PDOSet1 process data mapping.CPL28  sig_offset=10728  sig_type=uint16  type_size=16  sig_dim=1  device_id=0  sample_time=0.001000
      settings: SourceProductBaseCode=XP
  PDO Transmit CPL_CH29 : xpcethercatlib/EtherCAT PDO Transmit   Priority=3  sig_name=Box 4 (YISUWORLD_Dig).PDOSet1 process data mapping.CPL29  sig_offset=10744  sig_type=uint16  type_size=16  sig_dim=1  device_id=0  sample_time=0.001000
      settings: SourceProductBaseCode=XP
  PDO Transmit CPL_CH3 : xpcethercatlib/EtherCAT PDO Transmit   Priority=3  sig_name=Box 4 (YISUWORLD_Dig).PDOSet1 process data mapping.CPL3  sig_offset=10328  sig_type=uint16  type_size=16  sig_dim=1  device_id=0  sample_time=0.001000
      settings: SourceProductBaseCode=XP
  PDO Transmit CPL_CH30 : xpcethercatlib/EtherCAT PDO Transmit   Priority=3  sig_name=Box 4 (YISUWORLD_Dig).PDOSet1 process data mapping.CPL30  sig_offset=10760  sig_type=uint16  type_size=16  sig_dim=1  device_id=0  sample_time=0.001000
      settings: SourceProductBaseCode=XP
  PDO Transmit CPL_CH31 : xpcethercatlib/EtherCAT PDO Transmit   Priority=3  sig_name=Box 4 (YISUWORLD_Dig).PDOSet1 process data mapping.CPL31  sig_offset=10776  sig_type=uint16  type_size=16  sig_dim=1  device_id=0  sample_time=0.001000
      settings: SourceProductBaseCode=XP
  PDO Transmit CPL_CH32 : xpcethercatlib/EtherCAT PDO Transmit   Priority=3  sig_name=Box 4 (YISUWORLD_Dig).PDOSet1 process data mapping.CPL32  sig_offset=10792  sig_type=uint16  type_size=16  sig_dim=1  device_id=0  sample_time=0.001000
      settings: SourceProductBaseCode=XP
  PDO Transmit CPL_CH4 : xpcethercatlib/EtherCAT PDO Transmit   Priority=3  sig_name=Box 4 (YISUWORLD_Dig).PDOSet1 process data mapping.CPL4  sig_offset=10344  sig_type=uint16  type_size=16  sig_dim=1  device_id=0  sample_time=0.001000
      settings: SourceProductBaseCode=XP
  PDO Transmit CPL_CH5 : xpcethercatlib/EtherCAT PDO Transmit   Priority=3  sig_name=Box 4 (YISUWORLD_Dig).PDOSet1 process data mapping.CPL5  sig_offset=10360  sig_type=uint16  type_size=16  sig_dim=1  device_id=0  sample_time=0.001000
      settings: SourceProductBaseCode=XP
  PDO Transmit CPL_CH6 : xpcethercatlib/EtherCAT PDO Transmit   Priority=3  sig_name=Box 4 (YISUWORLD_Dig).PDOSet1 process data mapping.CPL6  sig_offset=10376  sig_type=uint16  type_size=16  sig_dim=1  device_id=0  sample_time=0.001000
      settings: SourceProductBaseCode=XP
  PDO Transmit CPL_CH7 : xpcethercatlib/EtherCAT PDO Transmit   Priority=3  sig_name=Box 4 (YISUWORLD_Dig).PDOSet1 process data mapping.CPL7  sig_offset=10392  sig_type=uint16  type_size=16  sig_dim=1  device_id=0  sample_time=0.001000
      settings: SourceProductBaseCode=XP
  PDO Transmit CPL_CH8 : xpcethercatlib/EtherCAT PDO Transmit   Priority=3  sig_name=Box 4 (YISUWORLD_Dig).PDOSet1 process data mapping.CPL8  sig_offset=10408  sig_type=uint16  type_size=16  sig_dim=1  device_id=0  sample_time=0.001000
      settings: SourceProductBaseCode=XP
  PDO Transmit CPL_CH9 : xpcethercatlib/EtherCAT PDO Transmit   Priority=3  sig_name=Box 4 (YISUWORLD_Dig).PDOSet1 process data mapping.CPL9  sig_offset=10424  sig_type=uint16  type_size=16  sig_dim=1  device_id=0  sample_time=0.001000
      settings: SourceProductBaseCode=XP
  PWM_CAP_CH{1..32} (32 alike) : yisutbxlib_utilities/PWM_CAP  SystemSampleTime=-1  Latency=0  AutoFrameSizeCalculation=off
      settings: SourceProductName=YISU Toolbox Library
  PWMCAP_DutyCycle_CH1 : Outport
  PWMCAP_Period_CH1 : Outport  Port=2
  PWMCAP_DutyCycle_CH2 : Outport  Port=3
  PWMCAP_Period_CH2 : Outport  Port=4
  PWMCAP_DutyCycle_CH3 : Outport  Port=5
  PWMCAP_Period_CH3 : Outport  Port=6
  PWMCAP_DutyCycle_CH4 : Outport  Port=7
  PWMCAP_Period_CH4 : Outport  Port=8
  PWMCAP_DutyCycle_CH5 : Outport  Port=9
  PWMCAP_Period_CH5 : Outport  Port=10
  PWMCAP_DutyCycle_CH6 : Outport  Port=11
  PWMCAP_Period_CH6 : Outport  Port=12
  PWMCAP_DutyCycle_CH7 : Outport  Port=13
  PWMCAP_Period_CH7 : Outport  Port=14
  PWMCAP_DutyCycle_CH8 : Outport  Port=15
  PWMCAP_Period_CH8 : Outport  Port=16
  PWMCAP_DutyCycle_CH9 : Outport  Port=17
  PWMCAP_Period_CH9 : Outport  Port=18
  PWMCAP_DutyCycle_CH10 : Outport  Port=19
  PWMCAP_Period_CH10 : Outport  Port=20
  PWMCAP_DutyCycle_CH11 : Outport  Port=21
  PWMCAP_Period_CH11 : Outport  Port=22
  PWMCAP_DutyCycle_CH12 : Outport  Port=23
  PWMCAP_Period_CH12 : Outport  Port=24
  PWMCAP_DutyCycle_CH13 : Outport  Port=25
  PWMCAP_Period_CH13 : Outport  Port=26
  PWMCAP_DutyCycle_CH14 : Outport  Port=27
  PWMCAP_Period_CH14 : Outport  Port=28
  PWMCAP_DutyCycle_CH15 : Outport  Port=29
  PWMCAP_Period_CH15 : Outport  Port=30
  PWMCAP_DutyCycle_CH16 : Outport  Port=31
  PWMCAP_Period_CH16 : Outport  Port=32
  PWMCAP_DutyCycle_CH17 : Outport  Port=33
  PWMCAP_Period_CH17 : Outport  Port=34
  PWMCAP_DutyCycle_CH18 : Outport  Port=35
  PWMCAP_Period_CH18 : Outport  Port=36
  PWMCAP_DutyCycle_CH19 : Outport  Port=37
  PWMCAP_Period_CH19 : Outport  Port=38
  PWMCAP_DutyCycle_CH20 : Outport  Port=39
  PWMCAP_Period_CH20 : Outport  Port=40
  PWMCAP_DutyCycle_CH21 : Outport  Port=41
  PWMCAP_Period_CH21 : Outport  Port=42
  PWMCAP_DutyCycle_CH22 : Outport  Port=43
  PWMCAP_Period_CH22 : Outport  Port=44
  PWMCAP_DutyCycle_CH23 : Outport  Port=45
  PWMCAP_Period_CH23 : Outport  Port=46
  PWMCAP_DutyCycle_CH24 : Outport  Port=47
  PWMCAP_Period_CH24 : Outport  Port=48
  PWMCAP_DutyCycle_CH25 : Outport  Port=49
  PWMCAP_Period_CH25 : Outport  Port=50
  PWMCAP_DutyCycle_CH26 : Outport  Port=51
  PWMCAP_Period_CH26 : Outport  Port=52
  PWMCAP_DutyCycle_CH27 : Outport  Port=53
  PWMCAP_Period_CH27 : Outport  Port=54
  PWMCAP_DutyCycle_CH28 : Outport  Port=55
  PWMCAP_Period_CH28 : Outport  Port=56
  PWMCAP_DutyCycle_CH29 : Outport  Port=57
  PWMCAP_Period_CH29 : Outport  Port=58
  PWMCAP_DutyCycle_CH30 : Outport  Port=59
  PWMCAP_Period_CH30 : Outport  Port=60
  PWMCAP_DutyCycle_CH31 : Outport  Port=61
  PWMCAP_Period_CH31 : Outport  Port=62
  PWMCAP_DutyCycle_CH32 : Outport  Port=63
  PWMCAP_Period_CH32 : Outport  Port=64
  wires:
  Constant CPL_CH1/1 -> DTCB CPL_CH1/1
  DTCB CPL_CH1/1 -> PDO Transmit CPL_CH1/1
  PDO Receive HTH_CH1/1 -> PWM_CAP_CH1/1
  PDO Receive HTL_CH1/1 -> PWM_CAP_CH1/2
  PDO Receive PH_CH1/1 -> PWM_CAP_CH1/3
  PDO Receive PL_CH1/1 -> PWM_CAP_CH1/4
  PWM_CAP_CH1/1 -> Gain_DC_CAP_CH1/1
  PWM_CAP_CH1/2 -> Gain_Period_CAP_CH1/1
  Gain_DC_CAP_CH1/1 -> PWMCAP_DutyCycle_CH1/1  "PWMCAP_DutyCycle_CH1"
  Gain_Period_CAP_CH1/1 -> PWMCAP_Period_CH1/1  "PWMCAP_Period_CH1"
  Constant CPL_CH2/1 -> DTCB CPL_CH2/1
  DTCB CPL_CH2/1 -> PDO Transmit CPL_CH2/1
  PDO Receive HTH_CH2/1 -> PWM_CAP_CH2/1
  PDO Receive HTL_CH2/1 -> PWM_CAP_CH2/2
  PDO Receive PH_CH2/1 -> PWM_CAP_CH2/3
  PDO Receive PL_CH2/1 -> PWM_CAP_CH2/4
  PWM_CAP_CH2/1 -> Gain_DC_CAP_CH2/1
  PWM_CAP_CH2/2 -> Gain_Period_CAP_CH2/1
  Gain_DC_CAP_CH2/1 -> PWMCAP_DutyCycle_CH2/1  "PWMCAP_DutyCycle_CH2"
  Gain_Period_CAP_CH2/1 -> PWMCAP_Period_CH2/1  "PWMCAP_Period_CH2"
  Constant CPL_CH3/1 -> DTCB CPL_CH3/1
  DTCB CPL_CH3/1 -> PDO Transmit CPL_CH3/1
  PDO Receive HTH_CH3/1 -> PWM_CAP_CH3/1
  PDO Receive HTL_CH3/1 -> PWM_CAP_CH3/2
  PDO Receive PH_CH3/1 -> PWM_CAP_CH3/3
  PDO Receive PL_CH3/1 -> PWM_CAP_CH3/4
  PWM_CAP_CH3/1 -> Gain_DC_CAP_CH3/1
  PWM_CAP_CH3/2 -> Gain_Period_CAP_CH3/1
  Gain_DC_CAP_CH3/1 -> PWMCAP_DutyCycle_CH3/1  "PWMCAP_DutyCycle_CH3"
  Gain_Period_CAP_CH3/1 -> PWMCAP_Period_CH3/1  "PWMCAP_Period_CH3"
  Constant CPL_CH4/1 -> DTCB CPL_CH4/1
  DTCB CPL_CH4/1 -> PDO Transmit CPL_CH4/1
  PDO Receive HTH_CH4/1 -> PWM_CAP_CH4/1
  PDO Receive HTL_CH4/1 -> PWM_CAP_CH4/2
  PDO Receive PH_CH4/1 -> PWM_CAP_CH4/3
  PDO Receive PL_CH4/1 -> PWM_CAP_CH4/4
  PWM_CAP_CH4/1 -> Gain_DC_CAP_CH4/1
  PWM_CAP_CH4/2 -> Gain_Period_CAP_CH4/1
  Gain_DC_CAP_CH4/1 -> PWMCAP_DutyCycle_CH4/1  "PWMCAP_DutyCycle_CH4"
  Gain_Period_CAP_CH4/1 -> PWMCAP_Period_CH4/1  "PWMCAP_Period_CH4"
  Constant CPL_CH5/1 -> DTCB CPL_CH5/1
  DTCB CPL_CH5/1 -> PDO Transmit CPL_CH5/1
  PDO Receive HTH_CH5/1 -> PWM_CAP_CH5/1
  PDO Receive HTL_CH5/1 -> PWM_CAP_CH5/2
  PDO Receive PH_CH5/1 -> PWM_CAP_CH5/3
  PDO Receive PL_CH5/1 -> PWM_CAP_CH5/4
  PWM_CAP_CH5/1 -> Gain_DC_CAP_CH5/1
  PWM_CAP_CH5/2 -> Gain_Period_CAP_CH5/1
  Gain_DC_CAP_CH5/1 -> PWMCAP_DutyCycle_CH5/1  "PWMCAP_DutyCycle_CH5"
  Gain_Period_CAP_CH5/1 -> PWMCAP_Period_CH5/1  "PWMCAP_Period_CH5"
  Constant CPL_CH6/1 -> DTCB CPL_CH6/1
  DTCB CPL_CH6/1 -> PDO Transmit CPL_CH6/1
  PDO Receive HTH_CH6/1 -> PWM_CAP_CH6/1
  PDO Receive HTL_CH6/1 -> PWM_CAP_CH6/2
  PDO Receive PH_CH6/1 -> PWM_CAP_CH6/3
  PDO Receive PL_CH6/1 -> PWM_CAP_CH6/4
  PWM_CAP_CH6/1 -> Gain_DC_CAP_CH6/1
  PWM_CAP_CH6/2 -> Gain_Period_CAP_CH6/1
  Gain_DC_CAP_CH6/1 -> PWMCAP_DutyCycle_CH6/1  "PWMCAP_DutyCycle_CH6"
  Gain_Period_CAP_CH6/1 -> PWMCAP_Period_CH6/1  "PWMCAP_Period_CH6"
  Constant CPL_CH7/1 -> DTCB CPL_CH7/1
  DTCB CPL_CH7/1 -> PDO Transmit CPL_CH7/1
  PDO Receive HTH_CH7/1 -> PWM_CAP_CH7/1
  PDO Receive HTL_CH7/1 -> PWM_CAP_CH7/2
  PDO Receive PH_CH7/1 -> PWM_CAP_CH7/3
  PDO Receive PL_CH7/1 -> PWM_CAP_CH7/4
  PWM_CAP_CH7/1 -> Gain_DC_CAP_CH7/1
  PWM_CAP_CH7/2 -> Gain_Period_CAP_CH7/1
  Gain_DC_CAP_CH7/1 -> PWMCAP_DutyCycle_CH7/1  "PWMCAP_DutyCycle_CH7"
  Gain_Period_CAP_CH7/1 -> PWMCAP_Period_CH7/1  "PWMCAP_Period_CH7"
  Constant CPL_CH8/1 -> DTCB CPL_CH8/1
  DTCB CPL_CH8/1 -> PDO Transmit CPL_CH8/1
  PDO Receive HTH_CH8/1 -> PWM_CAP_CH8/1
  PDO Receive HTL_CH8/1 -> PWM_CAP_CH8/2
  PDO Receive PH_CH8/1 -> PWM_CAP_CH8/3
  PDO Receive PL_CH8/1 -> PWM_CAP_CH8/4
  PWM_CAP_CH8/1 -> Gain_DC_CAP_CH8/1
  PWM_CAP_CH8/2 -> Gain_Period_CAP_CH8/1
  Gain_DC_CAP_CH8/1 -> PWMCAP_DutyCycle_CH8/1  "PWMCAP_DutyCycle_CH8"
  Gain_Period_CAP_CH8/1 -> PWMCAP_Period_CH8/1  "PWMCAP_Period_CH8"
  Constant CPL_CH9/1 -> DTCB CPL_CH9/1
  DTCB CPL_CH9/1 -> PDO Transmit CPL_CH9/1
  PDO Receive HTH_CH9/1 -> PWM_CAP_CH9/1
  PDO Receive HTL_CH9/1 -> PWM_CAP_CH9/2
  PDO Receive PH_CH9/1 -> PWM_CAP_CH9/3
  PDO Receive PL_CH9/1 -> PWM_CAP_CH9/4
  PWM_CAP_CH9/1 -> Gain_DC_CAP_CH9/1
  PWM_CAP_CH9/2 -> Gain_Period_CAP_CH9/1
  Gain_DC_CAP_CH9/1 -> PWMCAP_DutyCycle_CH9/1  "PWMCAP_DutyCycle_CH9"
  Gain_Period_CAP_CH9/1 -> PWMCAP_Period_CH9/1  "PWMCAP_Period_CH9"
  Constant CPL_CH10/1 -> DTCB CPL_CH10/1
  DTCB CPL_CH10/1 -> PDO Transmit CPL_CH10/1
  PDO Receive HTH_CH10/1 -> PWM_CAP_CH10/1
  PDO Receive HTL_CH10/1 -> PWM_CAP_CH10/2
  PDO Receive PH_CH10/1 -> PWM_CAP_CH10/3
  PDO Receive PL_CH10/1 -> PWM_CAP_CH10/4
  PWM_CAP_CH10/1 -> Gain_DC_CAP_CH10/1
  PWM_CAP_CH10/2 -> Gain_Period_CAP_CH10/1
  Gain_DC_CAP_CH10/1 -> PWMCAP_DutyCycle_CH10/1  "PWMCAP_DutyCycle_CH10"
  Gain_Period_CAP_CH10/1 -> PWMCAP_Period_CH10/1  "PWMCAP_Period_CH10"
  Constant CPL_CH11/1 -> DTCB CPL_CH11/1
  DTCB CPL_CH11/1 -> PDO Transmit CPL_CH11/1
  PDO Receive HTH_CH11/1 -> PWM_CAP_CH11/1
  PDO Receive HTL_CH11/1 -> PWM_CAP_CH11/2
  PDO Receive PH_CH11/1 -> PWM_CAP_CH11/3
  PDO Receive PL_CH11/1 -> PWM_CAP_CH11/4
  PWM_CAP_CH11/1 -> Gain_DC_CAP_CH11/1
  PWM_CAP_CH11/2 -> Gain_Period_CAP_CH11/1
  Gain_DC_CAP_CH11/1 -> PWMCAP_DutyCycle_CH11/1  "PWMCAP_DutyCycle_CH11"
  Gain_Period_CAP_CH11/1 -> PWMCAP_Period_CH11/1  "PWMCAP_Period_CH11"
  Constant CPL_CH12/1 -> DTCB CPL_CH12/1
  DTCB CPL_CH12/1 -> PDO Transmit CPL_CH12/1
  PDO Receive HTH_CH12/1 -> PWM_CAP_CH12/1
  PDO Receive HTL_CH12/1 -> PWM_CAP_CH12/2
  PDO Receive PH_CH12/1 -> PWM_CAP_CH12/3
  PDO Receive PL_CH12/1 -> PWM_CAP_CH12/4
  PWM_CAP_CH12/1 -> Gain_DC_CAP_CH12/1
  PWM_CAP_CH12/2 -> Gain_Period_CAP_CH12/1
  Gain_DC_CAP_CH12/1 -> PWMCAP_DutyCycle_CH12/1  "PWMCAP_DutyCycle_CH12"
  Gain_Period_CAP_CH12/1 -> PWMCAP_Period_CH12/1  "PWMCAP_Period_CH12"
  Constant CPL_CH13/1 -> DTCB CPL_CH13/1
  DTCB CPL_CH13/1 -> PDO Transmit CPL_CH13/1
  PDO Receive HTH_CH13/1 -> PWM_CAP_CH13/1
  PDO Receive HTL_CH13/1 -> PWM_CAP_CH13/2
  PDO Receive PH_CH13/1 -> PWM_CAP_CH13/3
  PDO Receive PL_CH13/1 -> PWM_CAP_CH13/4
  PWM_CAP_CH13/1 -> Gain_DC_CAP_CH13/1
  PWM_CAP_CH13/2 -> Gain_Period_CAP_CH13/1
  Gain_DC_CAP_CH13/1 -> PWMCAP_DutyCycle_CH13/1  "PWMCAP_DutyCycle_CH13"
  Gain_Period_CAP_CH13/1 -> PWMCAP_Period_CH13/1  "PWMCAP_Period_CH13"
  Constant CPL_CH14/1 -> DTCB CPL_CH14/1
  DTCB CPL_CH14/1 -> PDO Transmit CPL_CH14/1
  PDO Receive HTH_CH14/1 -> PWM_CAP_CH14/1
  PDO Receive HTL_CH14/1 -> PWM_CAP_CH14/2
  PDO Receive PH_CH14/1 -> PWM_CAP_CH14/3
  PDO Receive PL_CH14/1 -> PWM_CAP_CH14/4
  PWM_CAP_CH14/1 -> Gain_DC_CAP_CH14/1
  PWM_CAP_CH14/2 -> Gain_Period_CAP_CH14/1
  Gain_DC_CAP_CH14/1 -> PWMCAP_DutyCycle_CH14/1  "PWMCAP_DutyCycle_CH14"
  Gain_Period_CAP_CH14/1 -> PWMCAP_Period_CH14/1  "PWMCAP_Period_CH14"
  Constant CPL_CH15/1 -> DTCB CPL_CH15/1
  DTCB CPL_CH15/1 -> PDO Transmit CPL_CH15/1
  PDO Receive HTH_CH15/1 -> PWM_CAP_CH15/1
  PDO Receive HTL_CH15/1 -> PWM_CAP_CH15/2
  PDO Receive PH_CH15/1 -> PWM_CAP_CH15/3
  PDO Receive PL_CH15/1 -> PWM_CAP_CH15/4
  PWM_CAP_CH15/1 -> Gain_DC_CAP_CH15/1
  PWM_CAP_CH15/2 -> Gain_Period_CAP_CH15/1
  Gain_DC_CAP_CH15/1 -> PWMCAP_DutyCycle_CH15/1  "PWMCAP_DutyCycle_CH15"
  Gain_Period_CAP_CH15/1 -> PWMCAP_Period_CH15/1  "PWMCAP_Period_CH15"
  Constant CPL_CH16/1 -> DTCB CPL_CH16/1
  DTCB CPL_CH16/1 -> PDO Transmit CPL_CH16/1
  PDO Receive HTH_CH16/1 -> PWM_CAP_CH16/1
  PDO Receive HTL_CH16/1 -> PWM_CAP_CH16/2
  PDO Receive PH_CH16/1 -> PWM_CAP_CH16/3
  PDO Receive PL_CH16/1 -> PWM_CAP_CH16/4
  PWM_CAP_CH16/1 -> Gain_DC_CAP_CH16/1
  PWM_CAP_CH16/2 -> Gain_Period_CAP_CH16/1
  Gain_DC_CAP_CH16/1 -> PWMCAP_DutyCycle_CH16/1  "PWMCAP_DutyCycle_CH16"
  Gain_Period_CAP_CH16/1 -> PWMCAP_Period_CH16/1  "PWMCAP_Period_CH16"
  Constant CPL_CH17/1 -> DTCB CPL_CH17/1
  DTCB CPL_CH17/1 -> PDO Transmit CPL_CH17/1
  PDO Receive HTH_CH17/1 -> PWM_CAP_CH17/1
  PDO Receive HTL_CH17/1 -> PWM_CAP_CH17/2
  PDO Receive PH_CH17/1 -> PWM_CAP_CH17/3
  PDO Receive PL_CH17/1 -> PWM_CAP_CH17/4
  PWM_CAP_CH17/1 -> Gain_DC_CAP_CH17/1
  PWM_CAP_CH17/2 -> Gain_Period_CAP_CH17/1
  Gain_DC_CAP_CH17/1 -> PWMCAP_DutyCycle_CH17/1  "PWMCAP_DutyCycle_CH17"
  Gain_Period_CAP_CH17/1 -> PWMCAP_Period_CH17/1  "PWMCAP_Period_CH17"
  Constant CPL_CH18/1 -> DTCB CPL_CH18/1
  DTCB CPL_CH18/1 -> PDO Transmit CPL_CH18/1
  PDO Receive HTH_CH18/1 -> PWM_CAP_CH18/1
  PDO Receive HTL_CH18/1 -> PWM_CAP_CH18/2
  PDO Receive PH_CH18/1 -> PWM_CAP_CH18/3
  PDO Receive PL_CH18/1 -> PWM_CAP_CH18/4
  PWM_CAP_CH18/1 -> Gain_DC_CAP_CH18/1
  PWM_CAP_CH18/2 -> Gain_Period_CAP_CH18/1
  Gain_DC_CAP_CH18/1 -> PWMCAP_DutyCycle_CH18/1  "PWMCAP_DutyCycle_CH18"
  Gain_Period_CAP_CH18/1 -> PWMCAP_Period_CH18/1  "PWMCAP_Period_CH18"
  Constant CPL_CH19/1 -> DTCB CPL_CH19/1
  DTCB CPL_CH19/1 -> PDO Transmit CPL_CH19/1
  PDO Receive HTH_CH19/1 -> PWM_CAP_CH19/1
  PDO Receive HTL_CH19/1 -> PWM_CAP_CH19/2
  PDO Receive PH_CH19/1 -> PWM_CAP_CH19/3
  PDO Receive PL_CH19/1 -> PWM_CAP_CH19/4
  PWM_CAP_CH19/1 -> Gain_DC_CAP_CH19/1
  PWM_CAP_CH19/2 -> Gain_Period_CAP_CH19/1
  Gain_DC_CAP_CH19/1 -> PWMCAP_DutyCycle_CH19/1  "PWMCAP_DutyCycle_CH19"
  Gain_Period_CAP_CH19/1 -> PWMCAP_Period_CH19/1  "PWMCAP_Period_CH19"
  Constant CPL_CH20/1 -> DTCB CPL_CH20/1
  DTCB CPL_CH20/1 -> PDO Transmit CPL_CH20/1
  PDO Receive HTH_CH20/1 -> PWM_CAP_CH20/1
  PDO Receive HTL_CH20/1 -> PWM_CAP_CH20/2
  PDO Receive PH_CH20/1 -> PWM_CAP_CH20/3
  PDO Receive PL_CH20/1 -> PWM_CAP_CH20/4
  PWM_CAP_CH20/1 -> Gain_DC_CAP_CH20/1
  PWM_CAP_CH20/2 -> Gain_Period_CAP_CH20/1
  Gain_DC_CAP_CH20/1 -> PWMCAP_DutyCycle_CH20/1  "PWMCAP_DutyCycle_CH20"
  Gain_Period_CAP_CH20/1 -> PWMCAP_Period_CH20/1  "PWMCAP_Period_CH20"
  Constant CPL_CH21/1 -> DTCB CPL_CH21/1
  DTCB CPL_CH21/1 -> PDO Transmit CPL_CH21/1
  PDO Receive HTH_CH21/1 -> PWM_CAP_CH21/1
  PDO Receive HTL_CH21/1 -> PWM_CAP_CH21/2
  PDO Receive PH_CH21/1 -> PWM_CAP_CH21/3
  PDO Receive PL_CH21/1 -> PWM_CAP_CH21/4
  PWM_CAP_CH21/1 -> Gain_DC_CAP_CH21/1
  PWM_CAP_CH21/2 -> Gain_Period_CAP_CH21/1
  Gain_DC_CAP_CH21/1 -> PWMCAP_DutyCycle_CH21/1  "PWMCAP_DutyCycle_CH21"
  Gain_Period_CAP_CH21/1 -> PWMCAP_Period_CH21/1  "PWMCAP_Period_CH21"
  Constant CPL_CH22/1 -> DTCB CPL_CH22/1
  DTCB CPL_CH22/1 -> PDO Transmit CPL_CH22/1
  PDO Receive HTH_CH22/1 -> PWM_CAP_CH22/1
  PDO Receive HTL_CH22/1 -> PWM_CAP_CH22/2
  PDO Receive PH_CH22/1 -> PWM_CAP_CH22/3
  PDO Receive PL_CH22/1 -> PWM_CAP_CH22/4
  PWM_CAP_CH22/1 -> Gain_DC_CAP_CH22/1
  PWM_CAP_CH22/2 -> Gain_Period_CAP_CH22/1
  Gain_DC_CAP_CH22/1 -> PWMCAP_DutyCycle_CH22/1  "PWMCAP_DutyCycle_CH22"
  Gain_Period_CAP_CH22/1 -> PWMCAP_Period_CH22/1  "PWMCAP_Period_CH22"
  Constant CPL_CH23/1 -> DTCB CPL_CH23/1
  DTCB CPL_CH23/1 -> PDO Transmit CPL_CH23/1
  PDO Receive HTH_CH23/1 -> PWM_CAP_CH23/1
  PDO Receive HTL_CH23/1 -> PWM_CAP_CH23/2
  PDO Receive PH_CH23/1 -> PWM_CAP_CH23/3
  PDO Receive PL_CH23/1 -> PWM_CAP_CH23/4
  PWM_CAP_CH23/1 -> Gain_DC_CAP_CH23/1
  PWM_CAP_CH23/2 -> Gain_Period_CAP_CH23/1
  Gain_DC_CAP_CH23/1 -> PWMCAP_DutyCycle_CH23/1  "PWMCAP_DutyCycle_CH23"
  Gain_Period_CAP_CH23/1 -> PWMCAP_Period_CH23/1  "PWMCAP_Period_CH23"
  Constant CPL_CH24/1 -> DTCB CPL_CH24/1
  DTCB CPL_CH24/1 -> PDO Transmit CPL_CH24/1
  PDO Receive HTH_CH24/1 -> PWM_CAP_CH24/1
  PDO Receive HTL_CH24/1 -> PWM_CAP_CH24/2
  PDO Receive PH_CH24/1 -> PWM_CAP_CH24/3
  PDO Receive PL_CH24/1 -> PWM_CAP_CH24/4
  PWM_CAP_CH24/1 -> Gain_DC_CAP_CH24/1
  PWM_CAP_CH24/2 -> Gain_Period_CAP_CH24/1
  Gain_DC_CAP_CH24/1 -> PWMCAP_DutyCycle_CH24/1  "PWMCAP_DutyCycle_CH24"
  Gain_Period_CAP_CH24/1 -> PWMCAP_Period_CH24/1  "PWMCAP_Period_CH24"
  Constant CPL_CH25/1 -> DTCB CPL_CH25/1
  DTCB CPL_CH25/1 -> PDO Transmit CPL_CH25/1
  PDO Receive HTH_CH25/1 -> PWM_CAP_CH25/1
  PDO Receive HTL_CH25/1 -> PWM_CAP_CH25/2
  PDO Receive PH_CH25/1 -> PWM_CAP_CH25/3
  PDO Receive PL_CH25/1 -> PWM_CAP_CH25/4
  PWM_CAP_CH25/1 -> Gain_DC_CAP_CH25/1
  PWM_CAP_CH25/2 -> Gain_Period_CAP_CH25/1
  Gain_DC_CAP_CH25/1 -> PWMCAP_DutyCycle_CH25/1  "PWMCAP_DutyCycle_CH25"
  Gain_Period_CAP_CH25/1 -> PWMCAP_Period_CH25/1  "PWMCAP_Period_CH25"
  Constant CPL_CH26/1 -> DTCB CPL_CH26/1
  DTCB CPL_CH26/1 -> PDO Transmit CPL_CH26/1
  PDO Receive HTH_CH26/1 -> PWM_CAP_CH26/1
  PDO Receive HTL_CH26/1 -> PWM_CAP_CH26/2
  PDO Receive PH_CH26/1 -> PWM_CAP_CH26/3
  PDO Receive PL_CH26/1 -> PWM_CAP_CH26/4
  PWM_CAP_CH26/1 -> Gain_DC_CAP_CH26/1
  PWM_CAP_CH26/2 -> Gain_Period_CAP_CH26/1
  Gain_DC_CAP_CH26/1 -> PWMCAP_DutyCycle_CH26/1  "PWMCAP_DutyCycle_CH26"
  Gain_Period_CAP_CH26/1 -> PWMCAP_Period_CH26/1  "PWMCAP_Period_CH26"
  Constant CPL_CH27/1 -> DTCB CPL_CH27/1
  DTCB CPL_CH27/1 -> PDO Transmit CPL_CH27/1
  PDO Receive HTH_CH27/1 -> PWM_CAP_CH27/1
  PDO Receive HTL_CH27/1 -> PWM_CAP_CH27/2
  PDO Receive PH_CH27/1 -> PWM_CAP_CH27/3
  PDO Receive PL_CH27/1 -> PWM_CAP_CH27/4
  PWM_CAP_CH27/1 -> Gain_DC_CAP_CH27/1
  PWM_CAP_CH27/2 -> Gain_Period_CAP_CH27/1
  Gain_DC_CAP_CH27/1 -> PWMCAP_DutyCycle_CH27/1  "PWMCAP_DutyCycle_CH27"
  Gain_Period_CAP_CH27/1 -> PWMCAP_Period_CH27/1  "PWMCAP_Period_CH27"
  Constant CPL_CH28/1 -> DTCB CPL_CH28/1
  DTCB CPL_CH28/1 -> PDO Transmit CPL_CH28/1
  PDO Receive HTH_CH28/1 -> PWM_CAP_CH28/1
  PDO Receive HTL_CH28/1 -> PWM_CAP_CH28/2
  PDO Receive PH_CH28/1 -> PWM_CAP_CH28/3
  PDO Receive PL_CH28/1 -> PWM_CAP_CH28/4
  PWM_CAP_CH28/1 -> Gain_DC_CAP_CH28/1
  PWM_CAP_CH28/2 -> Gain_Period_CAP_CH28/1
  Gain_DC_CAP_CH28/1 -> PWMCAP_DutyCycle_CH28/1  "PWMCAP_DutyCycle_CH28"
  Gain_Period_CAP_CH28/1 -> PWMCAP_Period_CH28/1  "PWMCAP_Period_CH28"
  Constant CPL_CH29/1 -> DTCB CPL_CH29/1
  DTCB CPL_CH29/1 -> PDO Transmit CPL_CH29/1
  PDO Receive HTH_CH29/1 -> PWM_CAP_CH29/1
  PDO Receive HTL_CH29/1 -> PWM_CAP_CH29/2
  PDO Receive PH_CH29/1 -> PWM_CAP_CH29/3
  PDO Receive PL_CH29/1 -> PWM_CAP_CH29/4
  PWM_CAP_CH29/1 -> Gain_DC_CAP_CH29/1
  PWM_CAP_CH29/2 -> Gain_Period_CAP_CH29/1
  Gain_DC_CAP_CH29/1 -> PWMCAP_DutyCycle_CH29/1  "PWMCAP_DutyCycle_CH29"
  Gain_Period_CAP_CH29/1 -> PWMCAP_Period_CH29/1  "PWMCAP_Period_CH29"
  Constant CPL_CH30/1 -> DTCB CPL_CH30/1
  DTCB CPL_CH30/1 -> PDO Transmit CPL_CH30/1
  PDO Receive HTH_CH30/1 -> PWM_CAP_CH30/1
  PDO Receive HTL_CH30/1 -> PWM_CAP_CH30/2
  PDO Receive PH_CH30/1 -> PWM_CAP_CH30/3
  PDO Receive PL_CH30/1 -> PWM_CAP_CH30/4
  PWM_CAP_CH30/1 -> Gain_DC_CAP_CH30/1
  PWM_CAP_CH30/2 -> Gain_Period_CAP_CH30/1
  Gain_DC_CAP_CH30/1 -> PWMCAP_DutyCycle_CH30/1  "PWMCAP_DutyCycle_CH30"
  Gain_Period_CAP_CH30/1 -> PWMCAP_Period_CH30/1  "PWMCAP_Period_CH30"
  Constant CPL_CH31/1 -> DTCB CPL_CH31/1
  DTCB CPL_CH31/1 -> PDO Transmit CPL_CH31/1
  PDO Receive HTH_CH31/1 -> PWM_CAP_CH31/1
  PDO Receive HTL_CH31/1 -> PWM_CAP_CH31/2
  PDO Receive PH_CH31/1 -> PWM_CAP_CH31/3
  PDO Receive PL_CH31/1 -> PWM_CAP_CH31/4
  PWM_CAP_CH31/1 -> Gain_DC_CAP_CH31/1
  PWM_CAP_CH31/2 -> Gain_Period_CAP_CH31/1
  Gain_DC_CAP_CH31/1 -> PWMCAP_DutyCycle_CH31/1  "PWMCAP_DutyCycle_CH31"
  Gain_Period_CAP_CH31/1 -> PWMCAP_Period_CH31/1  "PWMCAP_Period_CH31"
  Constant CPL_CH32/1 -> DTCB CPL_CH32/1
  DTCB CPL_CH32/1 -> PDO Transmit CPL_CH32/1
  PDO Receive HTH_CH32/1 -> PWM_CAP_CH32/1
  PDO Receive HTL_CH32/1 -> PWM_CAP_CH32/2
  PDO Receive PH_CH32/1 -> PWM_CAP_CH32/3
  PDO Receive PL_CH32/1 -> PWM_CAP_CH32/4
  PWM_CAP_CH32/1 -> Gain_DC_CAP_CH32/1
  PWM_CAP_CH32/2 -> Gain_Period_CAP_CH32/1
  Gain_DC_CAP_CH32/1 -> PWMCAP_DutyCycle_CH32/1  "PWMCAP_DutyCycle_CH32"
  Gain_Period_CAP_CH32/1 -> PWMCAP_Period_CH32/1  "PWMCAP_Period_CH32"
